simulink model "sinetosquare"  (R2022b)
settings: Solver=VariableStepAuto  StartTime=0.0  StopTime=30  MaxStep=0.01  RelTol=1e-3
settings Model: Creator=Brigosha_Guest  LastModifiedBy=Brigosha_Guest

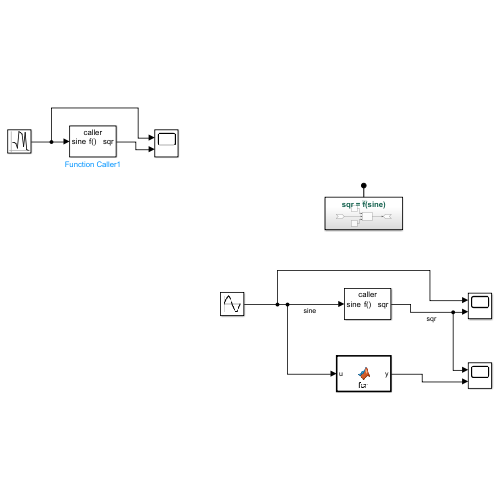
[thumbnail: Simulink's stored preview of the top-level diagram]
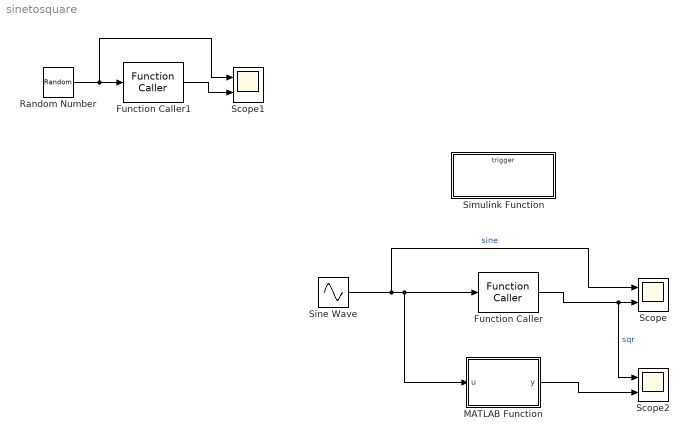
== system sinetosquare ==
  Function Caller : FunctionCaller  FunctionPrototype=sqr = f(sine)  InputArgumentSpecifications=<Enter example>  OutputArgumentSpecifications=<Enter example>
  Function Caller1 : FunctionCaller  FunctionPrototype=sqr = f(sine)  InputArgumentSpecifications=<Enter example>  OutputArgumentSpecifications=<Enter example>
  MATLAB Function : MATLAB Function  TreatAsAtomicUnit=on
  Random Number : RandomNumber  SampleTime=0.1
  Scope : Scope  NumInputPorts=2
  Scope1 : Scope  NumInputPorts=2
  Scope2 : Scope  NumInputPorts=2
  Simulink Function : Subsystem  TreatAsAtomicUnit=on
  Sine Wave : Sin  SampleTime=0
  wires:
  Sine Wave/1 -> MATLAB Function/1(u), Function Caller/1, Scope/1  "sine"
  Function Caller/1 -> Scope2/1, Scope/2  "sqr"
  Random Number/1 -> Scope1/1, Function Caller1/1
  Function Caller1/1 -> Scope1/2
  MATLAB Function/1(y) -> Scope2/2

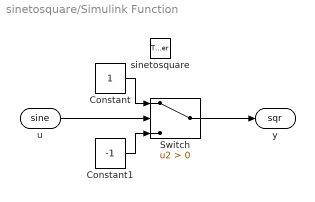
== system sinetosquare/Simulink Function ==
  sinetosquare : TriggerPort  TriggerType=function-call  IsSimulinkFunction=on  FunctionName=f  FunctionVisibility=scoped  VariantControl=(inherit)
  Constant : Constant
  Constant1 : Constant  Value=-1
  Switch : Switch  Criteria=u2 > Threshold  SaturateOnIntegerOverflow=off  InputSameDT=off
  u : ArgIn  DisableCoverage=on  ArgumentName=sine
  y : ArgOut  DisableCoverage=on  ArgumentName=sqr
  wires:
  u/1 -> Switch/2
  Constant/1 -> Switch/1
  Constant1/1 -> Switch/3
  Switch/1 -> y/1

== matlab function sinetosquare/MATLAB Function ==
  data: u input; y output
function y = fcn(u)
if u>0
    y=1;
else if u==0
        y=0;
else
    y=-1;
end
end
